simulink model "PMSM_controla"  (R2021a)
settings: Solver=VariableStepAuto  StartTime=0.0  StopTime=1  FixedStep=0.00001  MaxStep=1e-4  RelTol=1e-3
InitFcn:
  | Vdc=538
  | Tperiod = 0.001
  | 
  | r=1.2
  | Ld=5.7*10^-3
  | Lq=12.5*10^-3
  | PM=123*10^-3
  | P=4
  | b=0
  | J=0.0001
undefined symbols (not defined in the file): DiscIntNeverNeededParam
libraries: mcbcontrolslib x6, pid_lib x3
settings Model: Creator=Aliraqe  LastModifiedBy=Islam
settings SolverCC: AlgebraicLoopSolver=TrustRegion
settings DataIOCC: ReturnWorkspaceOutputs=off
settings DebuggingCC: SFMachineParentedDataDiag=warning  ArithmeticOperatorsInVariantConditions=warning
settings SFSimCC: SimUseLocalCustomCode=off  CustomCodeUndefinedFunction=UseInterfaceOnly
settings RTWCC: RTWUseLocalCustomCode=off

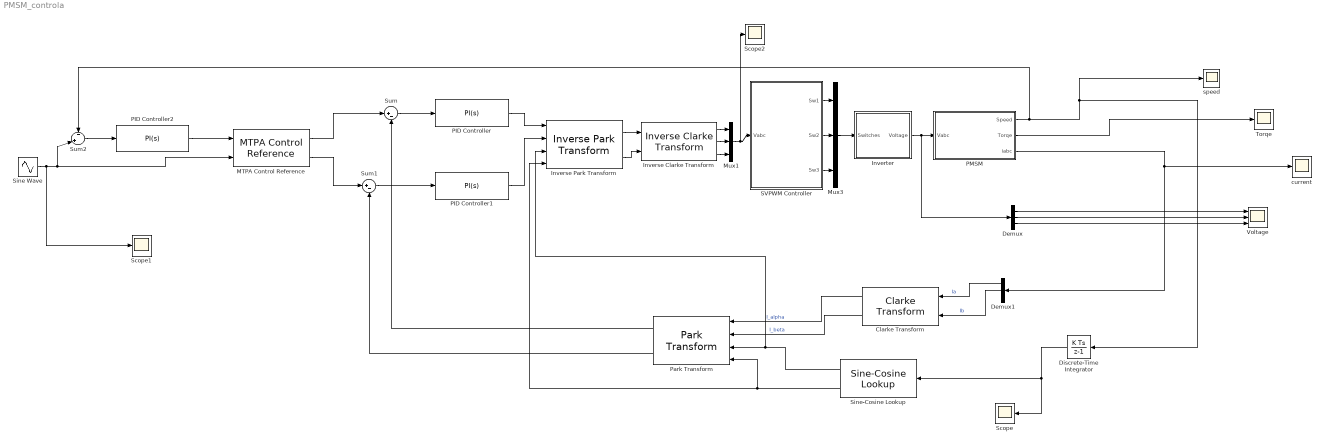
== system PMSM_controla ==
  Clarke Transform : mcbcontrolslib/Clarke Transform  VariantControl=Variant2
  Demux : Demux  Outputs=3
  Demux1 : Demux  Outputs=3
  Discrete-Time Integrator : DiscreteIntegrator  SampleTime=-1  ICPrevOutput=DiscIntNeverNeededParam  ICPrevScaledInput=DiscIntNeverNeededParam
  Inverse Clarke Transform : mcbcontrolslib/Inverse Clarke Transform
      settings: SourceProductBaseCode=MT
  Inverse Park Transform : mcbcontrolslib/Inverse Park Transform  AxisAlignment=D-axis
  "Inverter " : Subsystem
  MTPA Control Reference : mcbcontrolslib/MTPA Control Reference  LabelModeActiveChoice=Interior PMSM  VariantSelect=Interior PMSM  polePairs=4  Rs=0.36  Ld=0.2e-3  Lq=0.4e-3  FluxPM=6.4e-3  I_sat=7.1  V_dc=24  Units=Per-Unit (PU)  N_base=4107  I_base=19.3  T_base=0.74112  N_base_disp=3182
      settings: SourceProductBaseCode=MT
  Mux1 : Mux  Inputs=3
  Mux3 : Mux  Inputs=3
  PID Controller : pid_lib/PID Controller  Controller=PI  Form=Parallel  TimeDomain=Continuous-time  UseExternalTs=off  SampleTime=-1  IntegratorMethod=Forward Euler  FilterMethod=Forward Euler  ControllerParametersSource=internal  P=1  I=1  D=0  UseFilter=on  N=100  TunerSelectOption=Transfer Function Based (PID Tuner App)  InitialConditionSource=internal  InitialConditionForIntegrator=0  InitialConditionForFilter=0  DifferentiatorICPrevScaledInput=0  ExternalReset=none  TrackingMode=off  Kt=1  LimitOutput=off  SatLimitsSource=internal  UpperSaturationLimit=inf  LowerSaturationLimit=-inf  LinearizeAsGain=on  AntiWindupMode=none  Kb=1  POutMin=[]  POutMax=[]  IOutMin=[]  IOutMax=[]  DOutMin=[]  DOutMax=[]  NOutMin=[]  NOutMax=[]  SumOutMin=[]  SumOutMax=[]  SaturationOutMin=[]  SaturationOutMax=[]  PParamMin=[]  PParamMax=[]  IParamMin=[]  IParamMax=[]  DParamMin=[]  DParamMax=[]  NParamMin=[]  NParamMax=[]  KbParamMin=[]  KbParamMax=[]  KtParamMin=[]  KtParamMax=[]  KbOutMin=[]  KbOutMax=[]  KtOutMin=[]  KtOutMax=[]  IntegratorOutMin=[]  IntegratorOutMax=[]  FilterOutMin=[]  FilterOutMax=[]  SumI1OutMin=[]  SumI1OutMax=[]  SumI2OutMin=[]  SumI2OutMax=[]  SumI3OutMin=[]  SumI3OutMax=[]  SumI4OutMin=[]  SumI4OutMax=[]  SumDOutMin=[]  SumDOutMax=[]  DifferentiatorOutMin=[]  DifferentiatorOutMax=[]  FilterDiffOutCoefMin=[]  FilterDiffOutCoefMax=[]  ReciprocalOutMin=[]  ReciprocalOutMax=[]  SumDenOutMin=[]  SumDenOutMax=[]  SumNumOutMin=[]  SumNumOutMax=[]  DivideOutMin=[]  DivideOutMax=[]  UdiffTsProdOutMin=[]  UdiffTsProdOutMax=[]  NTsProdOutMin=[]  NTsProdOutMax=[]  UintegralTsProdOutMin=[]  UintegralTsProdOutMax=[]  UngainTsProdOutMin=[]  UngainTsProdOutMax=[]  IntegratorContinuousStateAttributes=''  IntegratorStateMustResolveToSignalObject=off  IntegratorRTWStateStorageClass=Auto  FilterContinuousStateAttributes=''  FilterStateMustResolveToSignalObject=off  FilterRTWStateStorageClass=Auto  ParallelPVariant=InternalParameters  IdealPVariant=Disabled  IVariant=InternalParameters  DVariant=Disabled  IntegratorVariant=Continuous  SatVariant=Disabled  AWVariant=Passthrough  PCopyVariant=Disabled  TRVariant=Disabled  FdbkBlocksVariant=Forward  IdealPFdbkVariant=Disabled  SatFdbkVariant=Disabled  DerivativeFilterVariant=Disabled  NVariant=Disabled  NCopyVariant=Disabled_SignalSpec  FilterICVariant=Disabled  IntegratorICVariant=InternalICs  ExternalResetVariant=Disabled  TRSumVariant=Passthrough  SumFdbkVariant=Disabled  SumVariant=Sum_PI  TsampFilterVariant=InternalTs  TsampNgainVariant=Passthrough  TsampIntegralVariant=Passthrough  ExternalSaturationOutDataTypeStr=Inherit: Same as second input
  PID Controller1 : pid_lib/PID Controller  Controller=PI  Form=Parallel  TimeDomain=Continuous-time  UseExternalTs=off  SampleTime=-1  IntegratorMethod=Forward Euler  FilterMethod=Forward Euler  ControllerParametersSource=internal  P=1  I=1  D=0  UseFilter=on  N=100  TunerSelectOption=Transfer Function Based (PID Tuner App)  InitialConditionSource=internal  InitialConditionForIntegrator=0  InitialConditionForFilter=0  DifferentiatorICPrevScaledInput=0  ExternalReset=none  TrackingMode=off  Kt=1  LimitOutput=off  SatLimitsSource=internal  UpperSaturationLimit=inf  LowerSaturationLimit=-inf  LinearizeAsGain=on  AntiWindupMode=none  Kb=1  POutMin=[]  POutMax=[]  IOutMin=[]  IOutMax=[]  DOutMin=[]  DOutMax=[]  NOutMin=[]  NOutMax=[]  SumOutMin=[]  SumOutMax=[]  SaturationOutMin=[]  SaturationOutMax=[]  PParamMin=[]  PParamMax=[]  IParamMin=[]  IParamMax=[]  DParamMin=[]  DParamMax=[]  NParamMin=[]  NParamMax=[]  KbParamMin=[]  KbParamMax=[]  KtParamMin=[]  KtParamMax=[]  KbOutMin=[]  KbOutMax=[]  KtOutMin=[]  KtOutMax=[]  IntegratorOutMin=[]  IntegratorOutMax=[]  FilterOutMin=[]  FilterOutMax=[]  SumI1OutMin=[]  SumI1OutMax=[]  SumI2OutMin=[]  SumI2OutMax=[]  SumI3OutMin=[]  SumI3OutMax=[]  SumI4OutMin=[]  SumI4OutMax=[]  SumDOutMin=[]  SumDOutMax=[]  DifferentiatorOutMin=[]  DifferentiatorOutMax=[]  FilterDiffOutCoefMin=[]  FilterDiffOutCoefMax=[]  ReciprocalOutMin=[]  ReciprocalOutMax=[]  SumDenOutMin=[]  SumDenOutMax=[]  SumNumOutMin=[]  SumNumOutMax=[]  DivideOutMin=[]  DivideOutMax=[]  UdiffTsProdOutMin=[]  UdiffTsProdOutMax=[]  NTsProdOutMin=[]  NTsProdOutMax=[]  UintegralTsProdOutMin=[]  UintegralTsProdOutMax=[]  UngainTsProdOutMin=[]  UngainTsProdOutMax=[]  IntegratorContinuousStateAttributes=''  IntegratorStateMustResolveToSignalObject=off  IntegratorRTWStateStorageClass=Auto  FilterContinuousStateAttributes=''  FilterStateMustResolveToSignalObject=off  FilterRTWStateStorageClass=Auto  ParallelPVariant=InternalParameters  IdealPVariant=Disabled  IVariant=InternalParameters  DVariant=Disabled  IntegratorVariant=Continuous  SatVariant=Disabled  AWVariant=Passthrough  PCopyVariant=Disabled  TRVariant=Disabled  FdbkBlocksVariant=Forward  IdealPFdbkVariant=Disabled  SatFdbkVariant=Disabled  DerivativeFilterVariant=Disabled  NVariant=Disabled  NCopyVariant=Disabled_SignalSpec  FilterICVariant=Disabled  IntegratorICVariant=InternalICs  ExternalResetVariant=Disabled  TRSumVariant=Passthrough  SumFdbkVariant=Disabled  SumVariant=Sum_PI  TsampFilterVariant=InternalTs  TsampNgainVariant=Passthrough  TsampIntegralVariant=Passthrough  ExternalSaturationOutDataTypeStr=Inherit: Same as second input
  PID Controller2 : pid_lib/PID Controller  Controller=PI  Form=Parallel  TimeDomain=Continuous-time  UseExternalTs=off  SampleTime=-1  IntegratorMethod=Forward Euler  FilterMethod=Forward Euler  ControllerParametersSource=internal  P=1  I=1  D=0  UseFilter=on  N=100  TunerSelectOption=Transfer Function Based (PID Tuner App)  InitialConditionSource=internal  InitialConditionForIntegrator=0  InitialConditionForFilter=0  DifferentiatorICPrevScaledInput=0  ExternalReset=none  TrackingMode=off  Kt=1  LimitOutput=off  SatLimitsSource=internal  UpperSaturationLimit=inf  LowerSaturationLimit=-inf  LinearizeAsGain=on  AntiWindupMode=none  Kb=1  POutMin=[]  POutMax=[]  IOutMin=[]  IOutMax=[]  DOutMin=[]  DOutMax=[]  NOutMin=[]  NOutMax=[]  SumOutMin=[]  SumOutMax=[]  SaturationOutMin=[]  SaturationOutMax=[]  PParamMin=[]  PParamMax=[]  IParamMin=[]  IParamMax=[]  DParamMin=[]  DParamMax=[]  NParamMin=[]  NParamMax=[]  KbParamMin=[]  KbParamMax=[]  KtParamMin=[]  KtParamMax=[]  KbOutMin=[]  KbOutMax=[]  KtOutMin=[]  KtOutMax=[]  IntegratorOutMin=[]  IntegratorOutMax=[]  FilterOutMin=[]  FilterOutMax=[]  SumI1OutMin=[]  SumI1OutMax=[]  SumI2OutMin=[]  SumI2OutMax=[]  SumI3OutMin=[]  SumI3OutMax=[]  SumI4OutMin=[]  SumI4OutMax=[]  SumDOutMin=[]  SumDOutMax=[]  DifferentiatorOutMin=[]  DifferentiatorOutMax=[]  FilterDiffOutCoefMin=[]  FilterDiffOutCoefMax=[]  ReciprocalOutMin=[]  ReciprocalOutMax=[]  SumDenOutMin=[]  SumDenOutMax=[]  SumNumOutMin=[]  SumNumOutMax=[]  DivideOutMin=[]  DivideOutMax=[]  UdiffTsProdOutMin=[]  UdiffTsProdOutMax=[]  NTsProdOutMin=[]  NTsProdOutMax=[]  UintegralTsProdOutMin=[]  UintegralTsProdOutMax=[]  UngainTsProdOutMin=[]  UngainTsProdOutMax=[]  IntegratorContinuousStateAttributes=''  IntegratorStateMustResolveToSignalObject=off  IntegratorRTWStateStorageClass=Auto  FilterContinuousStateAttributes=''  FilterStateMustResolveToSignalObject=off  FilterRTWStateStorageClass=Auto  ParallelPVariant=InternalParameters  IdealPVariant=Disabled  IVariant=InternalParameters  DVariant=Disabled  IntegratorVariant=Continuous  SatVariant=Disabled  AWVariant=Passthrough  PCopyVariant=Disabled  TRVariant=Disabled  FdbkBlocksVariant=Forward  IdealPFdbkVariant=Disabled  SatFdbkVariant=Disabled  DerivativeFilterVariant=Disabled  NVariant=Disabled  NCopyVariant=Disabled_SignalSpec  FilterICVariant=Disabled  IntegratorICVariant=InternalICs  ExternalResetVariant=Disabled  TRSumVariant=Passthrough  SumFdbkVariant=Disabled  SumVariant=Sum_PI  TsampFilterVariant=InternalTs  TsampNgainVariant=Passthrough  TsampIntegralVariant=Passthrough  ExternalSaturationOutDataTypeStr=Inherit: Same as second input
  PMSM : Subsystem
  Park Transform : mcbcontrolslib/Park Transform  AxisAlignment=D-axis
      settings: SourceProductBaseCode=MT
  SVPWM Controller : Subsystem
  Scope : Scope
  Scope1 : Scope
  Scope2 : Scope
  Sine Wave : Sin  Amplitude=0.5  Frequency=2  SampleTime=0
  Sine-Cosine Lookup : mcbcontrolslib/Sine-Cosine Lookup  AngleInput=Per-unit  N_points=1024
      settings: SourceProductBaseCode=MT
  Sum : Sum  Inputs=|+-
  Sum1 : Sum  Inputs=|+-
  Sum2 : Sum  Inputs=-|+|
  "Torqe " : Scope
  Voltage : Scope  NumInputPorts=3
  current : Scope
  speed : Scope
  wires:
  PMSM/2(Torqe) -> "Torqe "/1
  PMSM/1("Speed ") -> speed/1, Discrete-Time Integrator/1, Sum2/1
  PMSM/3(iabc) -> Demux1/1, current/1
  "Inverter "/1("Voltage ") -> Demux/1, PMSM/1(Vabc)
  SVPWM Controller/1(Sw1) -> Mux3/1
  SVPWM Controller/2(Sw2) -> Mux3/2
  SVPWM Controller/3(Sw3) -> Mux3/3
  Mux3/1 -> "Inverter "/1("Switches ")
  Demux/1 -> Voltage/1
  Demux/2 -> Voltage/2
  Demux/3 -> Voltage/3
  Clarke Transform/1 -> Park Transform/1  "I_alpha"
  Clarke Transform/2 -> Park Transform/2  "I_beta"
  Sine-Cosine Lookup/1 -> Inverse Park Transform/3, Park Transform/3
  Sine-Cosine Lookup/2 -> Inverse Park Transform/4, Park Transform/4
  Demux1/1 -> Clarke Transform/1  "Ia"
  Demux1/2 -> Clarke Transform/2  "Ib"
  Discrete-Time Integrator/1 -> Sine-Cosine Lookup/1, Scope/1
  Park Transform/1 -> Sum/2
  MTPA Control Reference/1 -> Sum/1
  Sum/1 -> PID Controller/1
  Sum1/1 -> PID Controller1/1
  Park Transform/2 -> Sum1/2
  MTPA Control Reference/2 -> Sum1/1
  PID Controller/1 -> Inverse Park Transform/1
  PID Controller1/1 -> Inverse Park Transform/2
  Inverse Park Transform/1 -> Inverse Clarke Transform/1
  Inverse Park Transform/2 -> Inverse Clarke Transform/2
  Inverse Clarke Transform/1 -> Mux1/1
  Inverse Clarke Transform/2 -> Mux1/2
  Inverse Clarke Transform/3 -> Mux1/3
  Mux1/1 -> Scope2/1, SVPWM Controller/1(Vabc)
  PID Controller2/1 -> MTPA Control Reference/1
  Sum2/1 -> PID Controller2/1
  Sine Wave/1 -> Scope1/1, MTPA Control Reference/2, Sum2/2

== system PMSM_controla/Inverter  ==
  "Switches " : Inport
  Fcn : Fcn  Expr=Vdc/3*(2*u(1)-u(2)-u(3))
  Fcn1 : Fcn  Expr=Vdc/3*(2*u(2)-u(1)-u(3))
  Fcn2 : Fcn  Expr=Vdc/3*(2*u(3)-u(2)-u(1))
  Mux1 : Mux  Inputs=3
  "Voltage " : Outport  VectorParamsAs1DForOutWhenUnconnected=off
  wires:
  Mux1/1 -> "Voltage "/1
  Fcn1/1 -> Mux1/2
  "Switches "/1 -> Fcn2/1, Fcn1/1, Fcn/1
  Fcn/1 -> Mux1/1
  Fcn2/1 -> Mux1/3

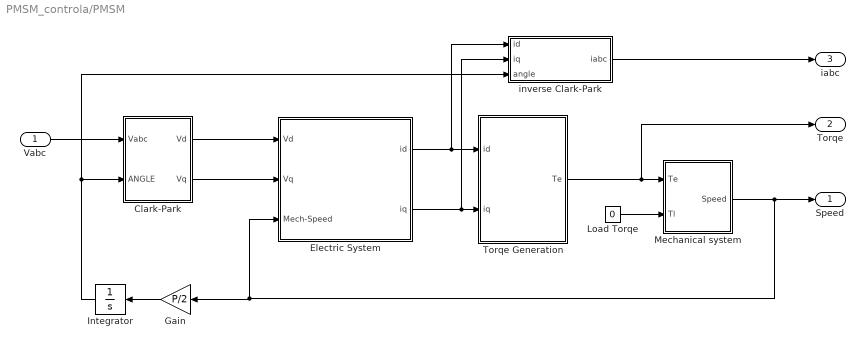
== system PMSM_controla/PMSM ==
  Vabc : Inport
  Clark-Park : Subsystem
  "Electric System " : Subsystem
  Gain : Gain  Gain=P/2
  Integrator : Integrator
  Load Torqe : Constant  Value=0
  Mechanical system : Subsystem
  Torqe Generation : Subsystem
  inverse Clark-Park : Subsystem
  "Speed " : Outport  VectorParamsAs1DForOutWhenUnconnected=off
  Torqe : Outport  Port=2  VectorParamsAs1DForOutWhenUnconnected=off
  iabc : Outport  Port=3  VectorParamsAs1DForOutWhenUnconnected=off
  wires:
  Load Torqe/1 -> Mechanical system/2(Tl)
  Clark-Park/1(Vd) -> "Electric System "/1(Vd)
  Torqe Generation/1(Te) -> Torqe/1, Mechanical system/1(Te)
  Clark-Park/2(Vq) -> "Electric System "/2("Vq ")
  Mechanical system/1(Speed) -> "Speed "/1, "Electric System "/3("Mech-Speed "), Gain/1
  "Electric System "/1("id ") -> Torqe Generation/1(id), inverse Clark-Park/1(id)
  Vabc/1 -> Clark-Park/1(Vabc)
  "Electric System "/2(iq) -> inverse Clark-Park/2(iq), Torqe Generation/2("iq ")
  Gain/1 -> Integrator/1
  Integrator/1 -> inverse Clark-Park/3(angle), Clark-Park/2("ANGLE ")
  inverse Clark-Park/1(iabc) -> iabc/1

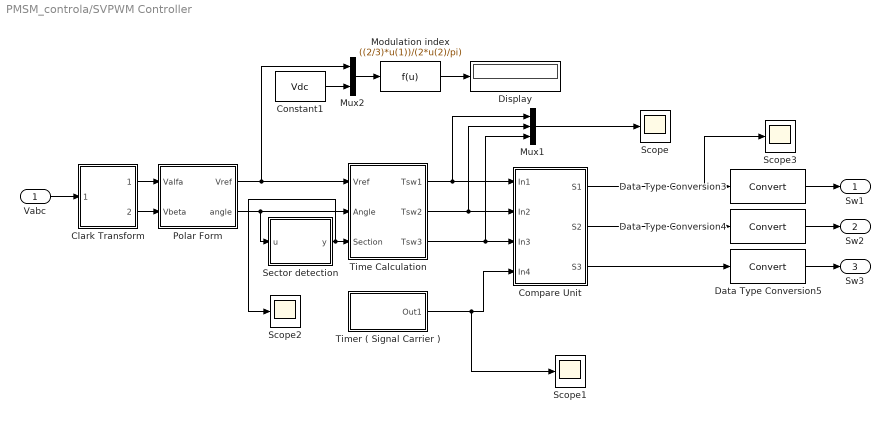
== system PMSM_controla/SVPWM Controller ==
  Vabc : Inport
  "Clark Transform " : Subsystem
  "Compare Unit " : Subsystem
  Constant1 : Constant  Value=Vdc
  Data Type Conversion3 : DataTypeConversion
  Data Type Conversion4 : DataTypeConversion
  Data Type Conversion5 : DataTypeConversion
  Display : Display
  Modulation index : Fcn  Expr=((2/3)*u(1))/(2*u(2)/pi)
  Mux1 : Mux  Inputs=3
  Mux2 : Mux  Inputs=2
  "Polar Form " : Subsystem
  Scope{,1..3} (4 alike) : Scope
  Sector detection : MATLAB Function  TreatAsAtomicUnit=on
  Time Calculation : Subsystem
  Timer ( Signal Carrier ) : Subsystem
  Sw1 : Outport  VectorParamsAs1DForOutWhenUnconnected=off
  Sw2 : Outport  Port=2  VectorParamsAs1DForOutWhenUnconnected=off
  Sw3 : Outport  Port=3  VectorParamsAs1DForOutWhenUnconnected=off
  wires:
  Mux1/1 -> Scope/1
  Time Calculation/3(Tsw3) -> Mux1/3, "Compare Unit "/3(In3)
  Time Calculation/2(Tsw2) -> Mux1/2, "Compare Unit "/2(In2)
  "Polar Form "/2(angle) -> Sector detection/1(u), Time Calculation/2(Angle)
  Sector detection/1(y) -> Scope2/1, Time Calculation/3(Section)
  "Clark Transform "/2(Vbeta) -> "Polar Form "/2(Vbeta)
  Time Calculation/1(Tsw1) -> Mux1/1, "Compare Unit "/1(In1)
  Vabc/1 -> "Clark Transform "/1("Vabc ")
  "Polar Form "/1(Vref) -> Time Calculation/1(Vref), Mux2/1
  Timer ( Signal Carrier )/1(Out1) -> Scope1/1, "Compare Unit "/4(In4)
  Mux2/1 -> Modulation index/1
  "Clark Transform "/1(Valfa) -> "Polar Form "/1(Valfa)
  Modulation index/1 -> Display/1
  Constant1/1 -> Mux2/2
  "Compare Unit "/3(S3) -> Data Type Conversion5/1
  "Compare Unit "/1(S1) -> Scope3/1, Data Type Conversion3/1
  "Compare Unit "/2(S2) -> Data Type Conversion4/1
  Data Type Conversion3/1 -> Sw1/1
  Data Type Conversion4/1 -> Sw2/1
  Data Type Conversion5/1 -> Sw3/1

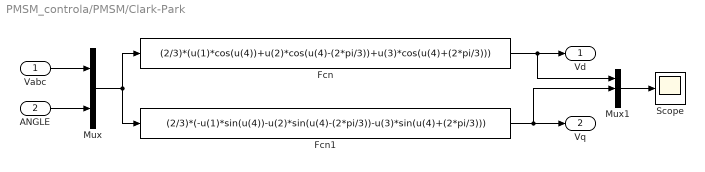
== system PMSM_controla/PMSM/Clark-Park ==
  Vabc : Inport
  "ANGLE " : Inport  Port=2
  Fcn : Fcn  Expr=(2/3)*(u(1)*cos(u(4))+u(2)*cos(u(4)-(2*pi/3))+u(3)*cos(u(4)+(2*pi/3)))
  Fcn1 : Fcn  Expr=(2/3)*(-u(1)*sin(u(4))-u(2)*sin(u(4)-(2*pi/3))-u(3)*sin(u(4)+(2*pi/3)))
  Mux : Mux  Inputs=2
  Mux1 : Mux  Inputs=3
  Scope : Scope
  Vd : Outport  VectorParamsAs1DForOutWhenUnconnected=off
  Vq : Outport  Port=2  VectorParamsAs1DForOutWhenUnconnected=off
  wires:
  Fcn/1 -> Mux1/1, Vd/1
  Vabc/1 -> Mux/1
  Mux/1 -> Fcn1/1, Fcn/1
  Fcn1/1 -> Mux1/2, Vq/1
  Mux1/1 -> Scope/1
  "ANGLE "/1 -> Mux/2

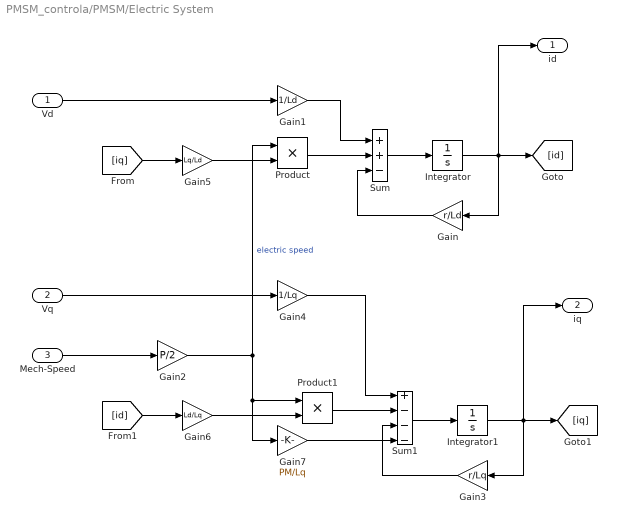
== system PMSM_controla/PMSM/Electric System  ==
  Vd : Inport
  "Vq " : Inport  Port=2
  "Mech-Speed " : Inport  Port=3
  Gain : Gain  Gain=r/Ld
  Gain1 : Gain  Gain=1/Ld
  Gain2 : Gain  Gain=P/2
  Gain3 : Gain  Gain=r/Lq
  Gain4 : Gain  Gain=1/Lq
  Gain5 : Gain  Gain=Lq/Ld
  Gain6 : Gain  Gain=Ld/Lq
  Gain7 : Gain  Gain=PM/Lq
  Integrator : Integrator
  Integrator1 : Integrator
  Product : Product
  Product1 : Product
  Sum : Sum  Inputs=++-
  Sum1 : Sum  Inputs=+---
  "id " : Outport  VectorParamsAs1DForOutWhenUnconnected=off
  iq : Outport  Port=2  VectorParamsAs1DForOutWhenUnconnected=off
  wires:
  Integrator/1 -> "id "/1, [id], Gain/1
  Gain1/1 -> Sum/1
  Sum/1 -> Integrator/1
  Vd/1 -> Gain1/1
  Gain/1 -> Sum/3
  Product/1 -> Sum/2
  Gain3/1 -> Sum1/3
  Gain4/1 -> Sum1/1
  Product1/1 -> Sum1/2
  "Vq "/1 -> Gain4/1
  Sum1/1 -> Integrator1/1
  Integrator1/1 -> iq/1, [iq], Gain3/1
  "Mech-Speed "/1 -> Gain2/1
  Gain2/1 -> Gain7/1, Product1/1, Product/1  "electric speed"
  [iq] -> Gain5/1
  Gain5/1 -> Product/2
  [id] -> Gain6/1
  Gain6/1 -> Product1/2
  Gain7/1 -> Sum1/4

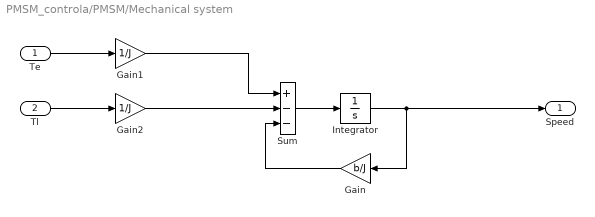
== system PMSM_controla/PMSM/Mechanical system ==
  Te : Inport
  Tl : Inport  Port=2
  Gain : Gain  Gain=b/J
  Gain1 : Gain  Gain=1/J
  Gain2 : Gain  Gain=1/J
  Integrator : Integrator
  Sum : Sum  Inputs=+--
  Speed : Outport  VectorParamsAs1DForOutWhenUnconnected=off
  wires:
  Integrator/1 -> Speed/1, Gain/1
  Gain1/1 -> Sum/1
  Gain2/1 -> Sum/2
  Sum/1 -> Integrator/1
  Gain/1 -> Sum/3
  Te/1 -> Gain1/1
  Tl/1 -> Gain2/1

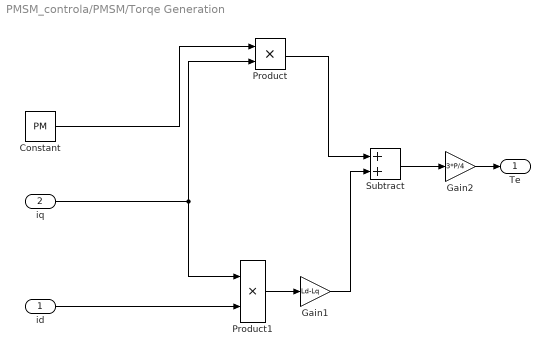
== system PMSM_controla/PMSM/Torqe Generation ==
  id : Inport
  "iq " : Inport  Port=2
  Constant : Constant  Value=PM
  Gain1 : Gain  Gain=Ld-Lq
  Gain2 : Gain  Gain=3*P/4
  Product : Product
  Product1 : Product
  Subtract : Sum
  Te : Outport  VectorParamsAs1DForOutWhenUnconnected=off
  wires:
  id/1 -> Product1/2
  Constant/1 -> Product/1
  "iq "/1 -> Product1/1, Product/2
  Product/1 -> Subtract/1
  Subtract/1 -> Gain2/1
  Gain2/1 -> Te/1
  Product1/1 -> Gain1/1
  Gain1/1 -> Subtract/2

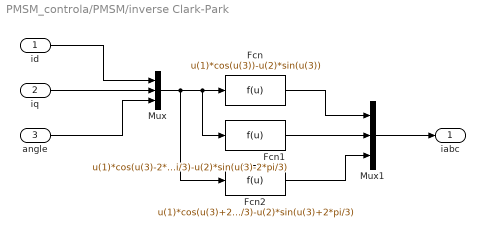
== system PMSM_controla/PMSM/inverse Clark-Park ==
  id : Inport
  iq : Inport  Port=2
  angle : Inport  Port=3
  Fcn : Fcn  Expr=u(1)*cos(u(3))-u(2)*sin(u(3))
  Fcn1 : Fcn  Expr=u(1)*cos(u(3)-2*pi/3)-u(2)*sin(u(3)-2*pi/3)
  Fcn2 : Fcn  Expr=u(1)*cos(u(3)+2*pi/3)-u(2)*sin(u(3)+2*pi/3)
  Mux : Mux  Inputs=3
  Mux1 : Mux  Inputs=3
  iabc : Outport  VectorParamsAs1DForOutWhenUnconnected=off
  wires:
  id/1 -> Mux/1
  iq/1 -> Mux/2
  angle/1 -> Mux/3
  Mux/1 -> Fcn2/1, Fcn1/1, Fcn/1
  Fcn/1 -> Mux1/1
  Fcn1/1 -> Mux1/2
  Fcn2/1 -> Mux1/3
  Mux1/1 -> iabc/1

== system PMSM_controla/SVPWM Controller/Clark Transform  ==
  "Vabc " : Inport
  Fcn : Fcn  Expr=(u(1)-1/2*u(2)-1/2*u(3))
  Fcn1 : Fcn  Expr=(0*u(1)+sqrt(3)/2*u(2)-sqrt(3)/2*u(3))
  Valfa : Outport  VectorParamsAs1DForOutWhenUnconnected=off
  Vbeta : Outport  Port=2  VectorParamsAs1DForOutWhenUnconnected=off
  wires:
  Fcn/1 -> Valfa/1
  "Vabc "/1 -> Fcn1/1, Fcn/1
  Fcn1/1 -> Vbeta/1

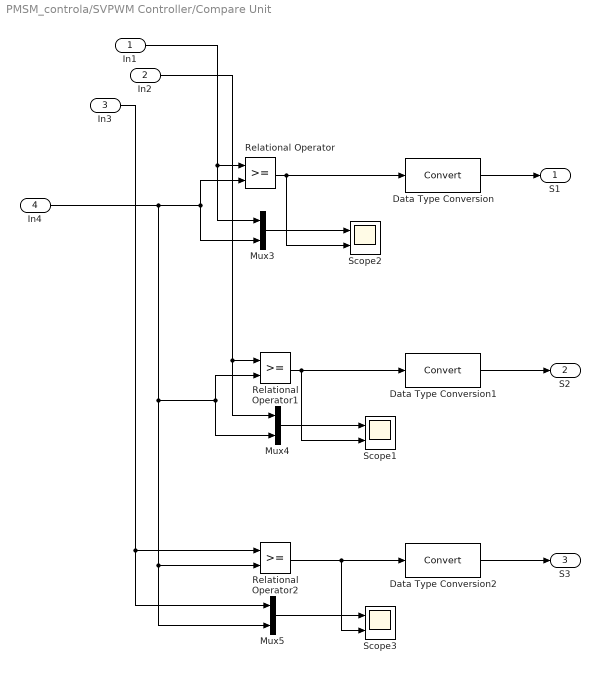
== system PMSM_controla/SVPWM Controller/Compare Unit  ==
  In1 : Inport
  In2 : Inport  Port=2
  In3 : Inport  Port=3
  In4 : Inport  Port=4
  Data Type Conversion : DataTypeConversion
  Data Type Conversion1 : DataTypeConversion
  Data Type Conversion2 : DataTypeConversion
  Mux3 : Mux  Inputs=2
  Mux4 : Mux  Inputs=2
  Mux5 : Mux  Inputs=2
  Relational Operator : RelationalOperator  OutDataTypeStr=boolean  RndMeth=Ceiling
  Relational Operator1 : RelationalOperator  OutDataTypeStr=boolean  RndMeth=Ceiling
  Relational Operator2 : RelationalOperator  OutDataTypeStr=boolean  RndMeth=Ceiling
  Scope1 : Scope  NumInputPorts=2
  Scope2 : Scope  NumInputPorts=2
  Scope3 : Scope  NumInputPorts=2
  S1 : Outport  VectorParamsAs1DForOutWhenUnconnected=off
  S2 : Outport  Port=2  VectorParamsAs1DForOutWhenUnconnected=off
  S3 : Outport  Port=3  VectorParamsAs1DForOutWhenUnconnected=off
  wires:
  Relational Operator/1 -> Data Type Conversion/1, Scope2/2
  In1/1 -> Relational Operator/1, Mux3/1
  In3/1 -> Relational Operator2/1, Mux5/1
  In2/1 -> Relational Operator1/1, Mux4/1
  Mux3/1 -> Scope2/1
  Mux4/1 -> Scope1/1
  Relational Operator1/1 -> Data Type Conversion1/1, Scope1/2
  Relational Operator2/1 -> Data Type Conversion2/1, Scope3/2
  Mux5/1 -> Scope3/1
  In4/1 -> Mux5/2, Relational Operator2/2, Mux4/2, Relational Operator1/2, Mux3/2, Relational Operator/2
  Data Type Conversion/1 -> S1/1
  Data Type Conversion1/1 -> S2/1
  Data Type Conversion2/1 -> S3/1

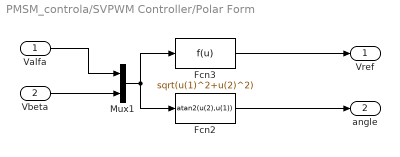
== system PMSM_controla/SVPWM Controller/Polar Form  ==
  Valfa : Inport
  Vbeta : Inport  Port=2
  Fcn2 : Fcn  Expr=atan2(u(2),u(1))
  Fcn3 : Fcn  Expr=sqrt(u(1)^2+u(2)^2)
  Mux1 : Mux  Inputs=2
  Vref : Outport  VectorParamsAs1DForOutWhenUnconnected=off
  angle : Outport  Port=2  VectorParamsAs1DForOutWhenUnconnected=off
  wires:
  Mux1/1 -> Fcn2/1, Fcn3/1
  Fcn3/1 -> Vref/1
  Valfa/1 -> Mux1/1
  Vbeta/1 -> Mux1/2
  Fcn2/1 -> angle/1

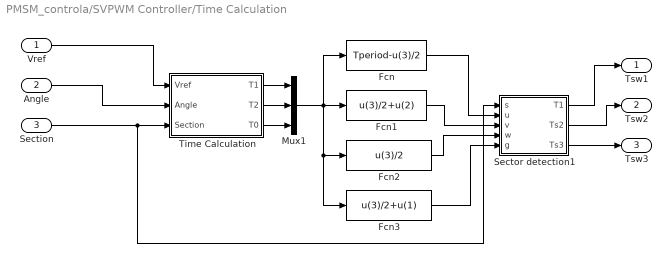
== system PMSM_controla/SVPWM Controller/Time Calculation ==
  Vref : Inport
  Angle : Inport  Port=2
  Section : Inport  Port=3
  Fcn : Fcn  Expr=Tperiod-u(3)/2
  Fcn1 : Fcn  Expr=u(3)/2+u(2)
  Fcn2 : Fcn  Expr=u(3)/2
  Fcn3 : Fcn  Expr=u(3)/2+u(1)
  Mux1 : Mux  Inputs=3
  Sector detection1 : MATLAB Function  TreatAsAtomicUnit=on
  Time Calculation : Subsystem
  Tsw1 : Outport  VectorParamsAs1DForOutWhenUnconnected=off
  Tsw2 : Outport  Port=2  VectorParamsAs1DForOutWhenUnconnected=off
  Tsw3 : Outport  Port=3  VectorParamsAs1DForOutWhenUnconnected=off
  wires:
  Time Calculation/1(T1) -> Mux1/1
  Sector detection1/1(T1) -> Tsw1/1
  Sector detection1/2(Ts2) -> Tsw2/1
  Vref/1 -> Time Calculation/1(Vref)
  Sector detection1/3(Ts3) -> Tsw3/1
  Angle/1 -> Time Calculation/2(Angle)
  Section/1 -> Sector detection1/1(s), Time Calculation/3(Section)
  Fcn2/1 -> Sector detection1/4(w)
  Fcn3/1 -> Sector detection1/5(g)
  Fcn1/1 -> Sector detection1/3(v)
  Mux1/1 -> Fcn/1, Fcn1/1, Fcn3/1, Fcn2/1
  Fcn/1 -> Sector detection1/2(u)
  Time Calculation/2(T2) -> Mux1/2
  Time Calculation/3(T0) -> Mux1/3

== system PMSM_controla/SVPWM Controller/Timer ( Signal Carrier ) ==
  Add : Sum
  Constant : Constant  Value=Tperiod
  Gain : Gain  Gain=1/Tperiod
  Integrator : Integrator
  Scope3 : Scope
  Signal Generator : SignalGenerator  WaveForm=square  Amplitude=Tperiod  Frequency=1/(2*Tperiod)
  Out1 : Outport  VectorParamsAs1DForOutWhenUnconnected=off
  wires:
  Add/1 -> Out1/1
  Gain/1 -> Add/1
  Signal Generator/1 -> Scope3/1, Integrator/1
  Integrator/1 -> Gain/1
  Constant/1 -> Add/2

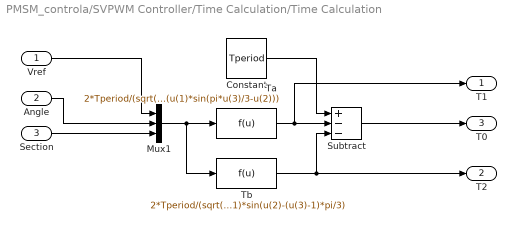
== system PMSM_controla/SVPWM Controller/Time Calculation/Time Calculation ==
  Vref : Inport
  Angle : Inport  Port=2
  Section : Inport  Port=3
  Constant : Constant  Value=Tperiod
  Mux1 : Mux  Inputs=3
  Subtract : Sum  Inputs=+--
  Ta : Fcn  Expr=2*Tperiod/(sqrt(3)*Vdc)*(u(1)*sin(pi*u(3)/3-u(2)))
  Tb : Fcn  Expr=2*Tperiod/(sqrt(3)*Vdc)*u(1)*sin(u(2)-(u(3)-1)*pi/3)
  T1 : Outport  VectorParamsAs1DForOutWhenUnconnected=off
  T2 : Outport  Port=2  VectorParamsAs1DForOutWhenUnconnected=off
  T0 : Outport  Port=3  VectorParamsAs1DForOutWhenUnconnected=off
  wires:
  Ta/1 -> Subtract/2, T1/1
  Mux1/1 -> Tb/1, Ta/1
  Vref/1 -> Mux1/1
  Angle/1 -> Mux1/2
  Section/1 -> Mux1/3
  Tb/1 -> T2/1, Subtract/3
  Constant/1 -> Subtract/1
  Subtract/1 -> T0/1

== matlab function PMSM_controla/SVPWM Controller/Time Calculation/Sector detection1 ==
  data: s input; u input; T1 output; v input; w input; g input; Ts2 output; Ts3 output
function [T1,Ts2,Ts3] = fcn(s,u,v,w,g)

switch s 
  
 case 1 
  T1 = u ; 
  Ts2 = v ;
  Ts3 = w ;
 case 2 
  T1 = g ; 
  Ts2 = u ; 
  Ts3 = w ;
 case 3 
  T1 = w ;
  Ts2 = u ; 
  Ts3 = v ; 
 case 4 
  T1 = w ;
  Ts2 = g ; 
  Ts3 = u ;
 case 5 
  T1 = v ;
  Ts2 = w ; 
  Ts3 = u ;
 case 6 
  T1 = u ;
  Ts2 = w ; 
  Ts3 = g ;
 otherwise 
 T1 = 0 ; 
 Ts2 = 0 ;
 Ts3 = 0 ;
 end 

end

== matlab function PMSM_controla/SVPWM Controller/Sector detection ==
  data: u input; y output
function y = fcn(u)

  u= 360/(2*pi)*u ; 
  
if (u>=0)&&(u<60)
  u = 1  ; 
elseif (u>=60)&&(u<120)
  u = 2  ;  
elseif (u>=120)&&(u<180)
  u = 3  ;  
elseif (u>=-180)&&(u<-120)
  u = 4  ;
elseif (u>=-120)&&(u<-60)
  u = 5  ;
elseif (u>=-60)&&(u<0)
  u = 6  ;
else
  u=0 ; 
end
y = u;
